simulink model "Sim_Ob_Edo"  (Simulink 10.3)
settings: Solver=VariableStepAuto  StartTime=0.0  StopTime=10.0  RelTol=1e-3  EnableMultiTasking=on
values from neighbouring files (symbols this model uses):
  Aco = [0 1 0 ... (first row only)    [Examen2PRetr_Edo.m]    (also in Retro_Edo.m = [-a1 1 0 0)
  bco = [ 0; 0; 1]    [Examen2PRetr_Edo.m]    (also in Retro_Edo.m = [0; 0; 0; 1])
  kco = T2*ko    [Examen2PRetr_Edo.m]
  T1 = MCc*inv(MCco)    [Examen2PRetr_Edo.m]
  T3 = inv(MOc)*MOo    [Examen2PRetr_Edo.m]
  vcero = zeros(3,1)    [CoOpt.m]    (also in Examen2PRetr_Edo.m; Retro_Edo.m)
  x0 = [1; 0; 0]    [CoOpt.m]    (also in Examen2PRetr_Edo.m = [-1; 0; 0]; Retro_Edo.m)
undefined symbols (not defined in the file or in its folder): Acok, I
settings Model: Creator=Tlayekanketl  LastModifiedBy=omarg
settings DataIOCC: LimitDataPoints=on
settings DebuggingCC: AllowSymbolicDim=off
settings ConfigComp: CovSFcnEnable=off

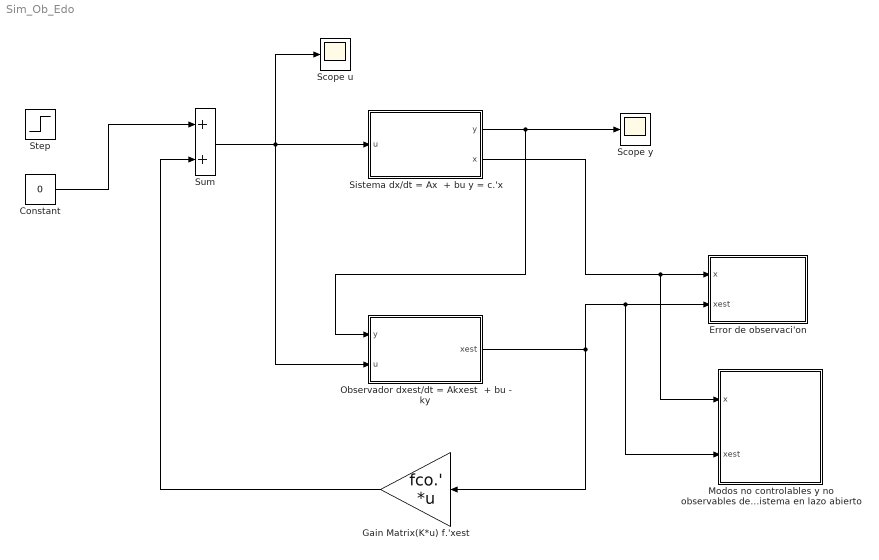
== system Sim_Ob_Edo ==
  Constant : Constant  Value=0
  Error de observaci'on : Subsystem
  Gain Matrix(K*u) f.'xest : Gain  Gain=fco.'  Multiplication=Matrix(K*u) (u vector)
  Modos no controlables y no observables del sistema en lazo abierto : Subsystem
  Observador dxest/dt = Akxest  + bu - ky : Subsystem
  Scope u : Scope
  Scope y : Scope
  Sistema dx/dt = Ax  + bu y = c.'x : Subsystem
  Step : Step  Time=0  SampleTime=0
  Sum : Sum
  wires:
  Sum/1 -> Sistema dx/dt = Ax  + bu y = c.'x/1(u), Observador dxest/dt = Akxest  + bu - ky/2(u), Scope u/1
  Gain Matrix(K*u) f.'xest/1 -> Sum/2
  Observador dxest/dt = Akxest  + bu - ky/1(xest) -> Gain Matrix(K*u) f.'xest/1, Error de observaci'on/2(xest), Modos no controlables y no observables del sistema en lazo abierto/2(xest)
  Sistema dx/dt = Ax  + bu y = c.'x/1(y) -> Scope y/1, Observador dxest/dt = Akxest  + bu - ky/1(y)
  Sistema dx/dt = Ax  + bu y = c.'x/2(x) -> Error de observaci'on/1(x), Modos no controlables y no observables del sistema en lazo abierto/1(x)
  Constant/1 -> Sum/1

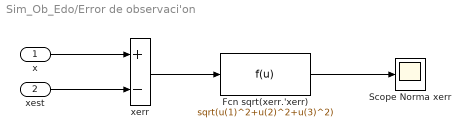
== system Sim_Ob_Edo/Error de observaci'on ==
  x : Inport
  xest : Inport  Port=2
  Fcn sqrt(xerr.'xerr) : Fcn  Expr=sqrt(u(1)^2+u(2)^2+u(3)^2)
  Scope Norma xerr : Scope
  xerr : Sum  Inputs=+-
  wires:
  xerr/1 -> Fcn sqrt(xerr.'xerr)/1
  Fcn sqrt(xerr.'xerr)/1 -> Scope Norma xerr/1
  xest/1 -> xerr/2
  x/1 -> xerr/1

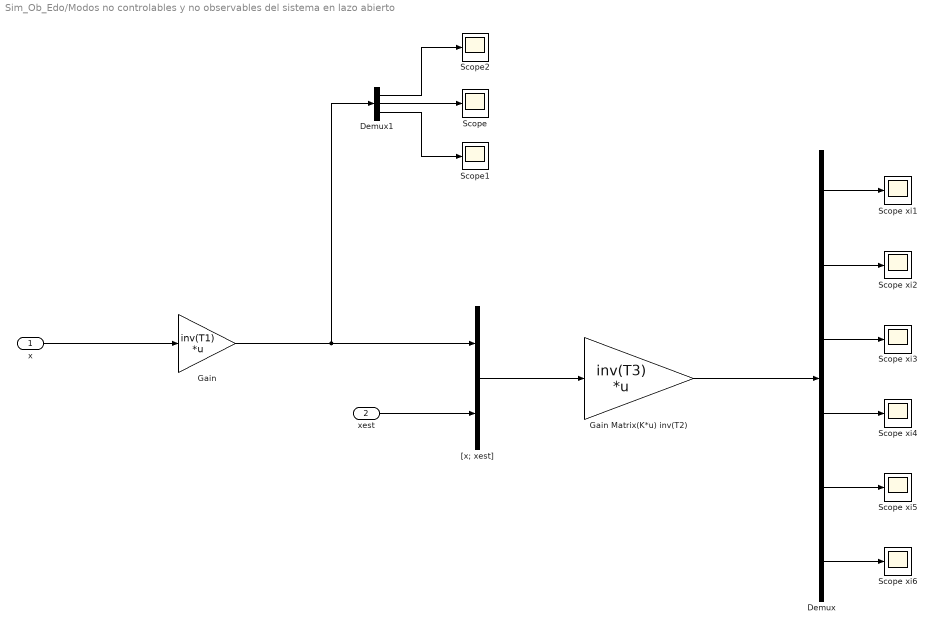
== system Sim_Ob_Edo/Modos no controlables y no observables del sistema en lazo abierto ==
  x : Inport
  xest : Inport  Port=2
  Demux : Demux  Outputs=6
  Demux1 : Demux  Outputs=3
  Gain : Gain  Gain=inv(T1)  Multiplication=Matrix(K*u) (u vector)
  Gain Matrix(K*u) inv(T2) : Gain  Gain=inv(T3)  Multiplication=Matrix(K*u) (u vector)
  Scope : Scope
  Scope xi{1..6} (6 alike) : Scope
  Scope1 : Scope
  Scope2 : Scope
  "[x; xest]" : Mux  Inputs=2
  wires:
  xest/1 -> "[x; xest]"/2
  "[x; xest]"/1 -> Gain Matrix(K*u) inv(T2)/1
  Demux/3 -> Scope xi3/1
  Demux/2 -> Scope xi2/1
  Demux/1 -> Scope xi1/1
  Demux/4 -> Scope xi4/1
  Demux/5 -> Scope xi5/1
  Demux/6 -> Scope xi6/1
  Gain Matrix(K*u) inv(T2)/1 -> Demux/1
  Demux1/1 -> Scope2/1
  Demux1/2 -> Scope/1
  Demux1/3 -> Scope1/1
  x/1 -> Gain/1
  Gain/1 -> Demux1/1, "[x; xest]"/1

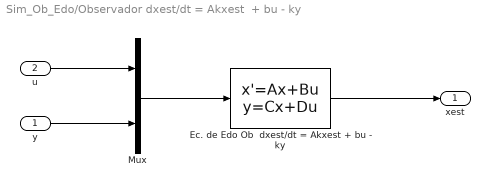
== system Sim_Ob_Edo/Observador dxest/dt = Akxest  + bu - ky ==
  y : Inport
  u : Inport  Port=2
  Ec. de Edo Ob  dxest/dt = Akxest + bu - ky : StateSpace  A=Acok  B=[bco -kco]  C=I  D=[vcero vcero]  InitialCondition=vcero
  Mux : Mux  Inputs=2
  xest : Outport
  wires:
  Mux/1 -> Ec. de Edo Ob  dxest/dt = Akxest + bu - ky/1
  Ec. de Edo Ob  dxest/dt = Akxest + bu - ky/1 -> xest/1
  u/1 -> Mux/1
  y/1 -> Mux/2

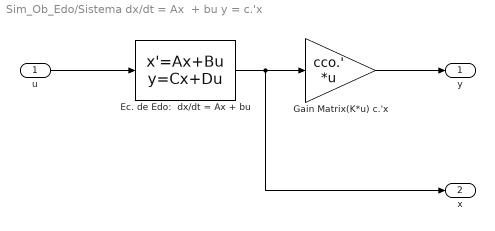
== system Sim_Ob_Edo/Sistema dx/dt = Ax  + bu y = c.'x ==
  u : Inport
  Ec. de Edo:  dx/dt = Ax + bu : StateSpace  A=Aco  B=bco  C=I  D=vcero  InitialCondition=x0
  Gain Matrix(K*u) c.'x : Gain  Gain=cco.'  Multiplication=Matrix(K*u) (u vector)
  y : Outport
  x : Outport  Port=2
  wires:
  u/1 -> Ec. de Edo:  dx/dt = Ax + bu/1
  Ec. de Edo:  dx/dt = Ax + bu/1 -> Gain Matrix(K*u) c.'x/1, x/1
  Gain Matrix(K*u) c.'x/1 -> y/1
